simulink model "uart_xy_wiggler"  (R2018a)
settings: Solver=FixedStepDiscrete  StartTime=0.0  StopTime=inf  RelTol=1e-3
PreLoadFcn:
  | waijung.modelPreload; % Required for working with Waijung Blockset. Do not remove.
undefined symbols (not defined in the file or in its folder): HSEOSC, Link, LQFP144, ST, STM32F446ZE
libraries: simulink x10, commsynccomp2 x7, stm32f4_io_lib x3, dspstat3 x2, stm32f4_device_config_lib x1, dspbuff3 x1
(part 8 of 9)

== system uart_xy_wiggler/set_UART_VCflag/Set UART vc Flag=6 ==
  UART Command : Inport
  Enable : EnablePort
  Volatile Data Storage Write : S-Function  FunctionName=waijung_vdata_write  Parameters=storagename,varname,sampletime,sampletimestr,blockid,storagetype,storagetypestr  SFunctionDeploymentMode=off  EnableBusSupport=off  mask(waijung_vdata_write){storagename=CircleR, varname=VolatileDataStorage7_CircleR, sampletime=.01, sampletimestr=-1, blockid=set_UART_VCflagSetUARTvcFlag6VolatileDataStorageWrite, storagetype=double, storagetypestr=double}
      mask prompts: storagename "Storage Name"; varname "Variable name"; sampletime "Sample time (sec)"; sampletimestr "Compiled sample time (sec) in string"; storagetype "Data type"; storagetypestr "Data type string"
      mask help: This block implements write data to a buffer.
      mask init:
      | waijung_vdata_write_callback('init');
      mask Help: web(fullfile(waijungdocroot,'Volatile_Data_Storage_Write.htm'))
      mask TypeOptions storagename: ab3 | ab1 | ab2 | ab4 | ab5 | ab6 | ab7 | ab8 | ab9 | ab10 | Ays | Ayc | Axs | A_Laser | LissaFreq | Axc | Laser | vcx | flag | CircleFlag | CircleFrequency | vcy | CircleR
      mask Callback storagename: waijung_vdata_write_callback('storagename');
      mask Callback varname: waijung_vdata_write_callback('varname');
      mask Callback sampletime: waijung_vdata_write_callback('sampletime');
      mask Callback sampletimestr: waijung_vdata_write_callback('sampletimestr');
      mask Callback blockid: waijung_vdata_write_callback('blockid');
      mask Callback storagetype: waijung_vdata_write_callback('storagetype');
      mask Display: text(0.95, 0.5, 'Buffer: CircleR','ver','middle','hor','right');port_label('input',1,'D1(double)')
  wires:
  UART Command/1 -> Volatile Data Storage Write/1

== system uart_xy_wiggler/set_UART_VCflag/flag_setting ==
  In1 : Inport
  Enable : EnablePort
  Data Type Conversion : DataTypeConversion
  Volatile Data Storage Write : S-Function  FunctionName=waijung_vdata_write  Parameters=storagename,varname,sampletime,sampletimestr,blockid,storagetype,storagetypestr  SFunctionDeploymentMode=off  EnableBusSupport=off  mask(waijung_vdata_write){storagename=flag, varname=VolatileDataStorage3_flag, sampletime=-1, sampletimestr=-1, blockid=set_UART_VCflagflag_settingVolatileDataStorageWrite, storagetype=uint8, storagetypestr=uint8_t}
      mask prompts: storagename "Storage Name"; varname "Variable name"; sampletime "Sample time (sec)"; sampletimestr "Compiled sample time (sec) in string"; storagetype "Data type"; storagetypestr "Data type string"
      mask help: This block implements write data to a buffer.
      mask init:
      | waijung_vdata_write_callback('init');
      mask Help: web(fullfile(waijungdocroot,'Volatile_Data_Storage_Write.htm'))
      mask TypeOptions storagename: ab3 | ab1 | ab2 | ab4 | ab5 | ab6 | ab7 | ab8 | ab9 | ab10 | Ays | Ayc | Axs | A_Laser | LissaFreq | Axc | Laser | vcx | flag | CircleFlag | CircleFrequency | vcy | CircleR
      mask Callback storagename: waijung_vdata_write_callback('storagename');
      mask Callback varname: waijung_vdata_write_callback('varname');
      mask Callback sampletime: waijung_vdata_write_callback('sampletime');
      mask Callback sampletimestr: waijung_vdata_write_callback('sampletimestr');
      mask Callback blockid: waijung_vdata_write_callback('blockid');
      mask Callback storagetype: waijung_vdata_write_callback('storagetype');
      mask Display: text(0.95, 0.5, 'Buffer: flag','ver','middle','hor','right');port_label('input',1,'D1(uint8)')
  wires:
  Data Type Conversion/1 -> Volatile Data Storage Write/1
  In1/1 -> Data Type Conversion/1

== system uart_xy_wiggler/Circle/Calibration Y/Subsystem1 ==
  Mux2 : Mux  Inputs=5
  Volatile Data Storage Read10 : S-Function  FunctionName=waijung_vdata_read  Parameters=storagename,varname,sampletime,sampletimestr,blockid,storagetype,storagetypestr  SFunctionDeploymentMode=off  EnableBusSupport=off  mask(waijung_vdata_read){storagename=ab10, varname=CalibrationDataVolatileDataStorage8_ab10, sampletime=.01, sampletimestr=-1, blockid=CircleCalibrationYSubsystem1VolatileDataStorageRead10, storagetype=double, storagetypestr=double}
      mask prompts: storagename "Storage Name"; varname "Variable name"; sampletime "Sample time (sec)"; sampletimestr "Compiled sample time (sec) in string"; storagetype "Data type"; storagetypestr "Data type string"
      mask help: This block implements read data from a buffer.
      mask init:
      | waijung_vdata_read_callback('init');
      mask Help: web(fullfile(waijungdocroot,'Volatile_Data_Storage_Read.htm'))
      mask TypeOptions storagename: ab3 | ab1 | ab2 | ab4 | ab5 | ab6 | ab7 | ab8 | ab9 | ab10 | Ays | Ayc | Axs | A_Laser | LissaFreq | Axc | Laser | vcx | flag | CircleFlag | CircleFrequency | vcy | CircleR
      mask Callback storagename: waijung_vdata_read_callback('storagename');
      mask Callback varname: waijung_vdata_read_callback('varname');
      mask Callback sampletime: waijung_vdata_read_callback('sampletime');
      mask Callback sampletimestr: waijung_vdata_read_callback('sampletimestr');
      mask Callback blockid: waijung_vdata_read_callback('blockid');
      mask Callback storagetype: waijung_vdata_read_callback('storagetype');
      mask Display: text(0.05, 0.5, 'Buffer: ab10','ver','middle','hor','left');port_label('output',1,'D1(double)')
  Volatile Data Storage Read6 : S-Function  FunctionName=waijung_vdata_read  Parameters=storagename,varname,sampletime,sampletimestr,blockid,storagetype,storagetypestr  SFunctionDeploymentMode=off  EnableBusSupport=off  mask(waijung_vdata_read){storagename=ab7, varname=CalibrationDataVolatileDataStorage5_ab7, sampletime=.01, sampletimestr=-1, blockid=CircleCalibrationYSubsystem1VolatileDataStorageRead6, storagetype=double, storagetypestr=double}
      mask prompts: storagename "Storage Name"; varname "Variable name"; sampletime "Sample time (sec)"; sampletimestr "Compiled sample time (sec) in string"; storagetype "Data type"; storagetypestr "Data type string"
      mask help: This block implements read data from a buffer.
      mask init:
      | waijung_vdata_read_callback('init');
      mask Help: web(fullfile(waijungdocroot,'Volatile_Data_Storage_Read.htm'))
      mask TypeOptions storagename: ab3 | ab1 | ab2 | ab4 | ab5 | ab6 | ab7 | ab8 | ab9 | ab10 | Ays | Ayc | Axs | A_Laser | LissaFreq | Axc | Laser | vcx | flag | CircleFlag | CircleFrequency | vcy | CircleR
      mask Callback storagename: waijung_vdata_read_callback('storagename');
      mask Callback varname: waijung_vdata_read_callback('varname');
      mask Callback sampletime: waijung_vdata_read_callback('sampletime');
      mask Callback sampletimestr: waijung_vdata_read_callback('sampletimestr');
      mask Callback blockid: waijung_vdata_read_callback('blockid');
      mask Callback storagetype: waijung_vdata_read_callback('storagetype');
      mask Display: text(0.05, 0.5, 'Buffer: ab7','ver','middle','hor','left');port_label('output',1,'D1(double)')
  Volatile Data Storage Read7 : S-Function  FunctionName=waijung_vdata_read  Parameters=storagename,varname,sampletime,sampletimestr,blockid,storagetype,storagetypestr  SFunctionDeploymentMode=off  EnableBusSupport=off  mask(waijung_vdata_read){storagename=ab8, varname=CalibrationDataVolatileDataStorage6_ab8, sampletime=.01, sampletimestr=-1, blockid=CircleCalibrationYSubsystem1VolatileDataStorageRead7, storagetype=double, storagetypestr=double}
      mask prompts: storagename "Storage Name"; varname "Variable name"; sampletime "Sample time (sec)"; sampletimestr "Compiled sample time (sec) in string"; storagetype "Data type"; storagetypestr "Data type string"
      mask help: This block implements read data from a buffer.
      mask init:
      | waijung_vdata_read_callback('init');
      mask Help: web(fullfile(waijungdocroot,'Volatile_Data_Storage_Read.htm'))
      mask TypeOptions storagename: ab3 | ab1 | ab2 | ab4 | ab5 | ab6 | ab7 | ab8 | ab9 | ab10 | Ays | Ayc | Axs | A_Laser | LissaFreq | Axc | Laser | vcx | flag | CircleFlag | CircleFrequency | vcy | CircleR
      mask Callback storagename: waijung_vdata_read_callback('storagename');
      mask Callback varname: waijung_vdata_read_callback('varname');
      mask Callback sampletime: waijung_vdata_read_callback('sampletime');
      mask Callback sampletimestr: waijung_vdata_read_callback('sampletimestr');
      mask Callback blockid: waijung_vdata_read_callback('blockid');
      mask Callback storagetype: waijung_vdata_read_callback('storagetype');
      mask Display: text(0.05, 0.5, 'Buffer: ab8','ver','middle','hor','left');port_label('output',1,'D1(double)')
  Volatile Data Storage Read8 : S-Function  FunctionName=waijung_vdata_read  Parameters=storagename,varname,sampletime,sampletimestr,blockid,storagetype,storagetypestr  SFunctionDeploymentMode=off  EnableBusSupport=off  mask(waijung_vdata_read){storagename=ab9, varname=CalibrationDataVolatileDataStorage7_ab9, sampletime=.01, sampletimestr=-1, blockid=CircleCalibrationYSubsystem1VolatileDataStorageRead8, storagetype=double, storagetypestr=double}
      mask prompts: storagename "Storage Name"; varname "Variable name"; sampletime "Sample time (sec)"; sampletimestr "Compiled sample time (sec) in string"; storagetype "Data type"; storagetypestr "Data type string"
      mask help: This block implements read data from a buffer.
      mask init:
      | waijung_vdata_read_callback('init');
      mask Help: web(fullfile(waijungdocroot,'Volatile_Data_Storage_Read.htm'))
      mask TypeOptions storagename: ab3 | ab1 | ab2 | ab4 | ab5 | ab6 | ab7 | ab8 | ab9 | ab10 | Ays | Ayc | Axs | A_Laser | LissaFreq | Axc | Laser | vcx | flag | CircleFlag | CircleFrequency | vcy | CircleR
      mask Callback storagename: waijung_vdata_read_callback('storagename');
      mask Callback varname: waijung_vdata_read_callback('varname');
      mask Callback sampletime: waijung_vdata_read_callback('sampletime');
      mask Callback sampletimestr: waijung_vdata_read_callback('sampletimestr');
      mask Callback blockid: waijung_vdata_read_callback('blockid');
      mask Callback storagetype: waijung_vdata_read_callback('storagetype');
      mask Display: text(0.05, 0.5, 'Buffer: ab9','ver','middle','hor','left');port_label('output',1,'D1(double)')
  Volatile Data Storage Read9 : S-Function  FunctionName=waijung_vdata_read  Parameters=storagename,varname,sampletime,sampletimestr,blockid,storagetype,storagetypestr  SFunctionDeploymentMode=off  EnableBusSupport=off  mask(waijung_vdata_read){storagename=ab6, varname=CalibrationDataVolatileDataStorage4_ab6, sampletime=.01, sampletimestr=-1, blockid=CircleCalibrationYSubsystem1VolatileDataStorageRead9, storagetype=double, storagetypestr=double}
      mask prompts: storagename "Storage Name"; varname "Variable name"; sampletime "Sample time (sec)"; sampletimestr "Compiled sample time (sec) in string"; storagetype "Data type"; storagetypestr "Data type string"
      mask help: This block implements read data from a buffer.
      mask init:
      | waijung_vdata_read_callback('init');
      mask Help: web(fullfile(waijungdocroot,'Volatile_Data_Storage_Read.htm'))
      mask TypeOptions storagename: ab3 | ab1 | ab2 | ab4 | ab5 | ab6 | ab7 | ab8 | ab9 | ab10 | Ays | Ayc | Axs | A_Laser | LissaFreq | Axc | Laser | vcx | flag | CircleFlag | CircleFrequency | vcy | CircleR
      mask Callback storagename: waijung_vdata_read_callback('storagename');
      mask Callback varname: waijung_vdata_read_callback('varname');
      mask Callback sampletime: waijung_vdata_read_callback('sampletime');
      mask Callback sampletimestr: waijung_vdata_read_callback('sampletimestr');
      mask Callback blockid: waijung_vdata_read_callback('blockid');
      mask Callback storagetype: waijung_vdata_read_callback('storagetype');
      mask Display: text(0.05, 0.5, 'Buffer: ab6','ver','middle','hor','left');port_label('output',1,'D1(double)')
  Y Calibration Coeff : Outport
  wires:
  Volatile Data Storage Read10/1 -> Mux2/5
  Volatile Data Storage Read8/1 -> Mux2/4
  Volatile Data Storage Read6/1 -> Mux2/2
  Volatile Data Storage Read7/1 -> Mux2/3
  Mux2/1 -> Y Calibration Coeff/1
  Volatile Data Storage Read9/1 -> Mux2/1

== system uart_xy_wiggler/Circle/Calibrtaion X/Subsystem ==
  Mux : Mux  Inputs=5
  Volatile Data Storage Read1 : S-Function  FunctionName=waijung_vdata_read  Parameters=storagename,varname,sampletime,sampletimestr,blockid,storagetype,storagetypestr  SFunctionDeploymentMode=off  EnableBusSupport=off  mask(waijung_vdata_read){storagename=ab2, varname=CalibrationDataVolatileDataStorage12_ab2, sampletime=.01, sampletimestr=-1, blockid=CircleCalibrtaionXSubsystemVolatileDataStorageRead1, storagetype=double, storagetypestr=double}
      mask prompts: storagename "Storage Name"; varname "Variable name"; sampletime "Sample time (sec)"; sampletimestr "Compiled sample time (sec) in string"; storagetype "Data type"; storagetypestr "Data type string"
      mask help: This block implements read data from a buffer.
      mask init:
      | waijung_vdata_read_callback('init');
      mask Help: web(fullfile(waijungdocroot,'Volatile_Data_Storage_Read.htm'))
      mask TypeOptions storagename: ab3 | ab1 | ab2 | ab4 | ab5 | ab6 | ab7 | ab8 | ab9 | ab10 | Ays | Ayc | Axs | A_Laser | LissaFreq | Axc | Laser | vcx | flag | CircleFlag | CircleFrequency | vcy | CircleR
      mask Callback storagename: waijung_vdata_read_callback('storagename');
      mask Callback varname: waijung_vdata_read_callback('varname');
      mask Callback sampletime: waijung_vdata_read_callback('sampletime');
      mask Callback sampletimestr: waijung_vdata_read_callback('sampletimestr');
      mask Callback blockid: waijung_vdata_read_callback('blockid');
      mask Callback storagetype: waijung_vdata_read_callback('storagetype');
      mask Display: text(0.05, 0.5, 'Buffer: ab2','ver','middle','hor','left');port_label('output',1,'D1(double)')
  Volatile Data Storage Read2 : S-Function  FunctionName=waijung_vdata_read  Parameters=storagename,varname,sampletime,sampletimestr,blockid,storagetype,storagetypestr  SFunctionDeploymentMode=off  EnableBusSupport=off  mask(waijung_vdata_read){storagename=ab3, varname=CalibrationDataVolatileDataStorage1_ab3, sampletime=.01, sampletimestr=-1, blockid=CircleCalibrtaionXSubsystemVolatileDataStorageRead2, storagetype=double, storagetypestr=double}
      mask prompts: storagename "Storage Name"; varname "Variable name"; sampletime "Sample time (sec)"; sampletimestr "Compiled sample time (sec) in string"; storagetype "Data type"; storagetypestr "Data type string"
      mask help: This block implements read data from a buffer.
      mask init:
      | waijung_vdata_read_callback('init');
      mask Help: web(fullfile(waijungdocroot,'Volatile_Data_Storage_Read.htm'))
      mask TypeOptions storagename: ab3 | ab1 | ab2 | ab4 | ab5 | ab6 | ab7 | ab8 | ab9 | ab10 | Ays | Ayc | Axs | A_Laser | LissaFreq | Axc | Laser | vcx | flag | CircleFlag | CircleFrequency | vcy | CircleR
      mask Callback storagename: waijung_vdata_read_callback('storagename');
      mask Callback varname: waijung_vdata_read_callback('varname');
      mask Callback sampletime: waijung_vdata_read_callback('sampletime');
      mask Callback sampletimestr: waijung_vdata_read_callback('sampletimestr');
      mask Callback blockid: waijung_vdata_read_callback('blockid');
      mask Callback storagetype: waijung_vdata_read_callback('storagetype');
      mask Display: text(0.05, 0.5, 'Buffer: ab3','ver','middle','hor','left');port_label('output',1,'D1(double)')
  Volatile Data Storage Read3 : S-Function  FunctionName=waijung_vdata_read  Parameters=storagename,varname,sampletime,sampletimestr,blockid,storagetype,storagetypestr  SFunctionDeploymentMode=off  EnableBusSupport=off  mask(waijung_vdata_read){storagename=ab4, varname=CalibrationDataVolatileDataStorage2_ab4, sampletime=.01, sampletimestr=-1, blockid=CircleCalibrtaionXSubsystemVolatileDataStorageRead3, storagetype=double, storagetypestr=double}
      mask prompts: storagename "Storage Name"; varname "Variable name"; sampletime "Sample time (sec)"; sampletimestr "Compiled sample time (sec) in string"; storagetype "Data type"; storagetypestr "Data type string"
      mask help: This block implements read data from a buffer.
      mask init:
      | waijung_vdata_read_callback('init');
      mask Help: web(fullfile(waijungdocroot,'Volatile_Data_Storage_Read.htm'))
      mask TypeOptions storagename: ab3 | ab1 | ab2 | ab4 | ab5 | ab6 | ab7 | ab8 | ab9 | ab10 | Ays | Ayc | Axs | A_Laser | LissaFreq | Axc | Laser | vcx | flag | CircleFlag | CircleFrequency | vcy | CircleR
      mask Callback storagename: waijung_vdata_read_callback('storagename');
      mask Callback varname: waijung_vdata_read_callback('varname');
      mask Callback sampletime: waijung_vdata_read_callback('sampletime');
      mask Callback sampletimestr: waijung_vdata_read_callback('sampletimestr');
      mask Callback blockid: waijung_vdata_read_callback('blockid');
      mask Callback storagetype: waijung_vdata_read_callback('storagetype');
      mask Display: text(0.05, 0.5, 'Buffer: ab4','ver','middle','hor','left');port_label('output',1,'D1(double)')
  Volatile Data Storage Read4 : S-Function  FunctionName=waijung_vdata_read  Parameters=storagename,varname,sampletime,sampletimestr,blockid,storagetype,storagetypestr  SFunctionDeploymentMode=off  EnableBusSupport=off  mask(waijung_vdata_read){storagename=ab1, varname=CalibrationDataVolatileDataStorage11_ab1, sampletime=.01, sampletimestr=-1, blockid=CircleCalibrtaionXSubsystemVolatileDataStorageRead4, storagetype=double, storagetypestr=double}
      mask prompts: storagename "Storage Name"; varname "Variable name"; sampletime "Sample time (sec)"; sampletimestr "Compiled sample time (sec) in string"; storagetype "Data type"; storagetypestr "Data type string"
      mask help: This block implements read data from a buffer.
      mask init:
      | waijung_vdata_read_callback('init');
      mask Help: web(fullfile(waijungdocroot,'Volatile_Data_Storage_Read.htm'))
      mask TypeOptions storagename: ab3 | ab1 | ab2 | ab4 | ab5 | ab6 | ab7 | ab8 | ab9 | ab10 | Ays | Ayc | Axs | A_Laser | LissaFreq | Axc | Laser | vcx | flag | CircleFlag | CircleFrequency | vcy | CircleR
      mask Callback storagename: waijung_vdata_read_callback('storagename');
      mask Callback varname: waijung_vdata_read_callback('varname');
      mask Callback sampletime: waijung_vdata_read_callback('sampletime');
      mask Callback sampletimestr: waijung_vdata_read_callback('sampletimestr');
      mask Callback blockid: waijung_vdata_read_callback('blockid');
      mask Callback storagetype: waijung_vdata_read_callback('storagetype');
      mask Display: text(0.05, 0.5, 'Buffer: ab1','ver','middle','hor','left');port_label('output',1,'D1(double)')
  Volatile Data Storage Read5 : S-Function  FunctionName=waijung_vdata_read  Parameters=storagename,varname,sampletime,sampletimestr,blockid,storagetype,storagetypestr  SFunctionDeploymentMode=off  EnableBusSupport=off  mask(waijung_vdata_read){storagename=ab5, varname=CalibrationDataVolatileDataStorage3_ab5, sampletime=.01, sampletimestr=-1, blockid=CircleCalibrtaionXSubsystemVolatileDataStorageRead5, storagetype=double, storagetypestr=double}
      mask prompts: storagename "Storage Name"; varname "Variable name"; sampletime "Sample time (sec)"; sampletimestr "Compiled sample time (sec) in string"; storagetype "Data type"; storagetypestr "Data type string"
      mask help: This block implements read data from a buffer.
      mask init:
      | waijung_vdata_read_callback('init');
      mask Help: web(fullfile(waijungdocroot,'Volatile_Data_Storage_Read.htm'))
      mask TypeOptions storagename: ab3 | ab1 | ab2 | ab4 | ab5 | ab6 | ab7 | ab8 | ab9 | ab10 | Ays | Ayc | Axs | A_Laser | LissaFreq | Axc | Laser | vcx | flag | CircleFlag | CircleFrequency | vcy | CircleR
      mask Callback storagename: waijung_vdata_read_callback('storagename');
      mask Callback varname: waijung_vdata_read_callback('varname');
      mask Callback sampletime: waijung_vdata_read_callback('sampletime');
      mask Callback sampletimestr: waijung_vdata_read_callback('sampletimestr');
      mask Callback blockid: waijung_vdata_read_callback('blockid');
      mask Callback storagetype: waijung_vdata_read_callback('storagetype');
      mask Display: text(0.05, 0.5, 'Buffer: ab5','ver','middle','hor','left');port_label('output',1,'D1(double)')
  X Calibration Coeff : Outport
  wires:
  Volatile Data Storage Read4/1 -> Mux/1
  Volatile Data Storage Read1/1 -> Mux/2
  Volatile Data Storage Read2/1 -> Mux/3
  Volatile Data Storage Read3/1 -> Mux/4
  Volatile Data Storage Read5/1 -> Mux/5
  Mux/1 -> X Calibration Coeff/1

== system uart_xy_wiggler/Lissajous/Calibration Y/Subsystem1 ==
  Mux2 : Mux  Inputs=5
  Volatile Data Storage Read10 : S-Function  FunctionName=waijung_vdata_read  Parameters=storagename,varname,sampletime,sampletimestr,blockid,storagetype,storagetypestr  SFunctionDeploymentMode=off  EnableBusSupport=off  mask(waijung_vdata_read){storagename=ab10, varname=CalibrationDataVolatileDataStorage8_ab10, sampletime=.01, sampletimestr=-1, blockid=LissajousCalibrationYSubsystem1VolatileDataStorageRead10, storagetype=double, storagetypestr=double}
      mask prompts: storagename "Storage Name"; varname "Variable name"; sampletime "Sample time (sec)"; sampletimestr "Compiled sample time (sec) in string"; storagetype "Data type"; storagetypestr "Data type string"
      mask help: This block implements read data from a buffer.
      mask init:
      | waijung_vdata_read_callback('init');
      mask Help: web(fullfile(waijungdocroot,'Volatile_Data_Storage_Read.htm'))
      mask TypeOptions storagename: ab3 | ab1 | ab2 | ab4 | ab5 | ab6 | ab7 | ab8 | ab9 | ab10 | Ays | Ayc | Axs | A_Laser | LissaFreq | Axc | Laser | vcx | flag | CircleFlag | CircleFrequency | vcy | CircleR
      mask Callback storagename: waijung_vdata_read_callback('storagename');
      mask Callback varname: waijung_vdata_read_callback('varname');
      mask Callback sampletime: waijung_vdata_read_callback('sampletime');
      mask Callback sampletimestr: waijung_vdata_read_callback('sampletimestr');
      mask Callback blockid: waijung_vdata_read_callback('blockid');
      mask Callback storagetype: waijung_vdata_read_callback('storagetype');
      mask Display: text(0.05, 0.5, 'Buffer: ab10','ver','middle','hor','left');port_label('output',1,'D1(double)')
  Volatile Data Storage Read6 : S-Function  FunctionName=waijung_vdata_read  Parameters=storagename,varname,sampletime,sampletimestr,blockid,storagetype,storagetypestr  SFunctionDeploymentMode=off  EnableBusSupport=off  mask(waijung_vdata_read){storagename=ab7, varname=CalibrationDataVolatileDataStorage5_ab7, sampletime=.01, sampletimestr=-1, blockid=LissajousCalibrationYSubsystem1VolatileDataStorageRead6, storagetype=double, storagetypestr=double}
      mask prompts: storagename "Storage Name"; varname "Variable name"; sampletime "Sample time (sec)"; sampletimestr "Compiled sample time (sec) in string"; storagetype "Data type"; storagetypestr "Data type string"
      mask help: This block implements read data from a buffer.
      mask init:
      | waijung_vdata_read_callback('init');
      mask Help: web(fullfile(waijungdocroot,'Volatile_Data_Storage_Read.htm'))
      mask TypeOptions storagename: ab3 | ab1 | ab2 | ab4 | ab5 | ab6 | ab7 | ab8 | ab9 | ab10 | Ays | Ayc | Axs | A_Laser | LissaFreq | Axc | Laser | vcx | flag | CircleFlag | CircleFrequency | vcy | CircleR
      mask Callback storagename: waijung_vdata_read_callback('storagename');
      mask Callback varname: waijung_vdata_read_callback('varname');
      mask Callback sampletime: waijung_vdata_read_callback('sampletime');
      mask Callback sampletimestr: waijung_vdata_read_callback('sampletimestr');
      mask Callback blockid: waijung_vdata_read_callback('blockid');
      mask Callback storagetype: waijung_vdata_read_callback('storagetype');
      mask Display: text(0.05, 0.5, 'Buffer: ab7','ver','middle','hor','left');port_label('output',1,'D1(double)')
  Volatile Data Storage Read7 : S-Function  FunctionName=waijung_vdata_read  Parameters=storagename,varname,sampletime,sampletimestr,blockid,storagetype,storagetypestr  SFunctionDeploymentMode=off  EnableBusSupport=off  mask(waijung_vdata_read){storagename=ab8, varname=CalibrationDataVolatileDataStorage6_ab8, sampletime=.01, sampletimestr=-1, blockid=LissajousCalibrationYSubsystem1VolatileDataStorageRead7, storagetype=double, storagetypestr=double}
      mask prompts: storagename "Storage Name"; varname "Variable name"; sampletime "Sample time (sec)"; sampletimestr "Compiled sample time (sec) in string"; storagetype "Data type"; storagetypestr "Data type string"
      mask help: This block implements read data from a buffer.
      mask init:
      | waijung_vdata_read_callback('init');
      mask Help: web(fullfile(waijungdocroot,'Volatile_Data_Storage_Read.htm'))
      mask TypeOptions storagename: ab3 | ab1 | ab2 | ab4 | ab5 | ab6 | ab7 | ab8 | ab9 | ab10 | Ays | Ayc | Axs | A_Laser | LissaFreq | Axc | Laser | vcx | flag | CircleFlag | CircleFrequency | vcy | CircleR
      mask Callback storagename: waijung_vdata_read_callback('storagename');
      mask Callback varname: waijung_vdata_read_callback('varname');
      mask Callback sampletime: waijung_vdata_read_callback('sampletime');
      mask Callback sampletimestr: waijung_vdata_read_callback('sampletimestr');
      mask Callback blockid: waijung_vdata_read_callback('blockid');
      mask Callback storagetype: waijung_vdata_read_callback('storagetype');
      mask Display: text(0.05, 0.5, 'Buffer: ab8','ver','middle','hor','left');port_label('output',1,'D1(double)')
  Volatile Data Storage Read8 : S-Function  FunctionName=waijung_vdata_read  Parameters=storagename,varname,sampletime,sampletimestr,blockid,storagetype,storagetypestr  SFunctionDeploymentMode=off  EnableBusSupport=off  mask(waijung_vdata_read){storagename=ab9, varname=CalibrationDataVolatileDataStorage7_ab9, sampletime=.01, sampletimestr=-1, blockid=LissajousCalibrationYSubsystem1VolatileDataStorageRead8, storagetype=double, storagetypestr=double}
      mask prompts: storagename "Storage Name"; varname "Variable name"; sampletime "Sample time (sec)"; sampletimestr "Compiled sample time (sec) in string"; storagetype "Data type"; storagetypestr "Data type string"
      mask help: This block implements read data from a buffer.
      mask init:
      | waijung_vdata_read_callback('init');
      mask Help: web(fullfile(waijungdocroot,'Volatile_Data_Storage_Read.htm'))
      mask TypeOptions storagename: ab3 | ab1 | ab2 | ab4 | ab5 | ab6 | ab7 | ab8 | ab9 | ab10 | Ays | Ayc | Axs | A_Laser | LissaFreq | Axc | Laser | vcx | flag | CircleFlag | CircleFrequency | vcy | CircleR
      mask Callback storagename: waijung_vdata_read_callback('storagename');
      mask Callback varname: waijung_vdata_read_callback('varname');
      mask Callback sampletime: waijung_vdata_read_callback('sampletime');
      mask Callback sampletimestr: waijung_vdata_read_callback('sampletimestr');
      mask Callback blockid: waijung_vdata_read_callback('blockid');
      mask Callback storagetype: waijung_vdata_read_callback('storagetype');
      mask Display: text(0.05, 0.5, 'Buffer: ab9','ver','middle','hor','left');port_label('output',1,'D1(double)')
  Volatile Data Storage Read9 : S-Function  FunctionName=waijung_vdata_read  Parameters=storagename,varname,sampletime,sampletimestr,blockid,storagetype,storagetypestr  SFunctionDeploymentMode=off  EnableBusSupport=off  mask(waijung_vdata_read){storagename=ab6, varname=CalibrationDataVolatileDataStorage4_ab6, sampletime=.01, sampletimestr=-1, blockid=LissajousCalibrationYSubsystem1VolatileDataStorageRead9, storagetype=double, storagetypestr=double}
      mask prompts: storagename "Storage Name"; varname "Variable name"; sampletime "Sample time (sec)"; sampletimestr "Compiled sample time (sec) in string"; storagetype "Data type"; storagetypestr "Data type string"
      mask help: This block implements read data from a buffer.
      mask init:
      | waijung_vdata_read_callback('init');
      mask Help: web(fullfile(waijungdocroot,'Volatile_Data_Storage_Read.htm'))
      mask TypeOptions storagename: ab3 | ab1 | ab2 | ab4 | ab5 | ab6 | ab7 | ab8 | ab9 | ab10 | Ays | Ayc | Axs | A_Laser | LissaFreq | Axc | Laser | vcx | flag | CircleFlag | CircleFrequency | vcy | CircleR
      mask Callback storagename: waijung_vdata_read_callback('storagename');
      mask Callback varname: waijung_vdata_read_callback('varname');
      mask Callback sampletime: waijung_vdata_read_callback('sampletime');
      mask Callback sampletimestr: waijung_vdata_read_callback('sampletimestr');
      mask Callback blockid: waijung_vdata_read_callback('blockid');
      mask Callback storagetype: waijung_vdata_read_callback('storagetype');
      mask Display: text(0.05, 0.5, 'Buffer: ab6','ver','middle','hor','left');port_label('output',1,'D1(double)')
  Y Calibration Coeff : Outport
  wires:
  Volatile Data Storage Read10/1 -> Mux2/5
  Volatile Data Storage Read8/1 -> Mux2/4
  Volatile Data Storage Read6/1 -> Mux2/2
  Volatile Data Storage Read7/1 -> Mux2/3
  Mux2/1 -> Y Calibration Coeff/1
  Volatile Data Storage Read9/1 -> Mux2/1

== system uart_xy_wiggler/Lissajous/Calibrtaion X/Subsystem ==
  Mux : Mux  Inputs=5
  Volatile Data Storage Read1 : S-Function  FunctionName=waijung_vdata_read  Parameters=storagename,varname,sampletime,sampletimestr,blockid,storagetype,storagetypestr  SFunctionDeploymentMode=off  EnableBusSupport=off  mask(waijung_vdata_read){storagename=ab2, varname=CalibrationDataVolatileDataStorage12_ab2, sampletime=.01, sampletimestr=-1, blockid=LissajousCalibrtaionXSubsystemVolatileDataStorageRead1, storagetype=double, storagetypestr=double}
      mask prompts: storagename "Storage Name"; varname "Variable name"; sampletime "Sample time (sec)"; sampletimestr "Compiled sample time (sec) in string"; storagetype "Data type"; storagetypestr "Data type string"
      mask help: This block implements read data from a buffer.
      mask init:
      | waijung_vdata_read_callback('init');
      mask Help: web(fullfile(waijungdocroot,'Volatile_Data_Storage_Read.htm'))
      mask TypeOptions storagename: ab3 | ab1 | ab2 | ab4 | ab5 | ab6 | ab7 | ab8 | ab9 | ab10 | Ays | Ayc | Axs | A_Laser | LissaFreq | Axc | Laser | vcx | flag | CircleFlag | CircleFrequency | vcy | CircleR
      mask Callback storagename: waijung_vdata_read_callback('storagename');
      mask Callback varname: waijung_vdata_read_callback('varname');
      mask Callback sampletime: waijung_vdata_read_callback('sampletime');
      mask Callback sampletimestr: waijung_vdata_read_callback('sampletimestr');
      mask Callback blockid: waijung_vdata_read_callback('blockid');
      mask Callback storagetype: waijung_vdata_read_callback('storagetype');
      mask Display: text(0.05, 0.5, 'Buffer: ab2','ver','middle','hor','left');port_label('output',1,'D1(double)')
  Volatile Data Storage Read2 : S-Function  FunctionName=waijung_vdata_read  Parameters=storagename,varname,sampletime,sampletimestr,blockid,storagetype,storagetypestr  SFunctionDeploymentMode=off  EnableBusSupport=off  mask(waijung_vdata_read){storagename=ab3, varname=CalibrationDataVolatileDataStorage1_ab3, sampletime=.01, sampletimestr=-1, blockid=LissajousCalibrtaionXSubsystemVolatileDataStorageRead2, storagetype=double, storagetypestr=double}
      mask prompts: storagename "Storage Name"; varname "Variable name"; sampletime "Sample time (sec)"; sampletimestr "Compiled sample time (sec) in string"; storagetype "Data type"; storagetypestr "Data type string"
      mask help: This block implements read data from a buffer.
      mask init:
      | waijung_vdata_read_callback('init');
      mask Help: web(fullfile(waijungdocroot,'Volatile_Data_Storage_Read.htm'))
      mask TypeOptions storagename: ab3 | ab1 | ab2 | ab4 | ab5 | ab6 | ab7 | ab8 | ab9 | ab10 | Ays | Ayc | Axs | A_Laser | LissaFreq | Axc | Laser | vcx | flag | CircleFlag | CircleFrequency | vcy | CircleR
      mask Callback storagename: waijung_vdata_read_callback('storagename');
      mask Callback varname: waijung_vdata_read_callback('varname');
      mask Callback sampletime: waijung_vdata_read_callback('sampletime');
      mask Callback sampletimestr: waijung_vdata_read_callback('sampletimestr');
      mask Callback blockid: waijung_vdata_read_callback('blockid');
      mask Callback storagetype: waijung_vdata_read_callback('storagetype');
      mask Display: text(0.05, 0.5, 'Buffer: ab3','ver','middle','hor','left');port_label('output',1,'D1(double)')
  Volatile Data Storage Read3 : S-Function  FunctionName=waijung_vdata_read  Parameters=storagename,varname,sampletime,sampletimestr,blockid,storagetype,storagetypestr  SFunctionDeploymentMode=off  EnableBusSupport=off  mask(waijung_vdata_read){storagename=ab4, varname=CalibrationDataVolatileDataStorage2_ab4, sampletime=.01, sampletimestr=-1, blockid=LissajousCalibrtaionXSubsystemVolatileDataStorageRead3, storagetype=double, storagetypestr=double}
      mask prompts: storagename "Storage Name"; varname "Variable name"; sampletime "Sample time (sec)"; sampletimestr "Compiled sample time (sec) in string"; storagetype "Data type"; storagetypestr "Data type string"
      mask help: This block implements read data from a buffer.
      mask init:
      | waijung_vdata_read_callback('init');
      mask Help: web(fullfile(waijungdocroot,'Volatile_Data_Storage_Read.htm'))
      mask TypeOptions storagename: ab3 | ab1 | ab2 | ab4 | ab5 | ab6 | ab7 | ab8 | ab9 | ab10 | Ays | Ayc | Axs | A_Laser | LissaFreq | Axc | Laser | vcx | flag | CircleFlag | CircleFrequency | vcy | CircleR
      mask Callback storagename: waijung_vdata_read_callback('storagename');
      mask Callback varname: waijung_vdata_read_callback('varname');
      mask Callback sampletime: waijung_vdata_read_callback('sampletime');
      mask Callback sampletimestr: waijung_vdata_read_callback('sampletimestr');
      mask Callback blockid: waijung_vdata_read_callback('blockid');
      mask Callback storagetype: waijung_vdata_read_callback('storagetype');
      mask Display: text(0.05, 0.5, 'Buffer: ab4','ver','middle','hor','left');port_label('output',1,'D1(double)')
  Volatile Data Storage Read4 : S-Function  FunctionName=waijung_vdata_read  Parameters=storagename,varname,sampletime,sampletimestr,blockid,storagetype,storagetypestr  SFunctionDeploymentMode=off  EnableBusSupport=off  mask(waijung_vdata_read){storagename=ab1, varname=CalibrationDataVolatileDataStorage11_ab1, sampletime=.01, sampletimestr=-1, blockid=LissajousCalibrtaionXSubsystemVolatileDataStorageRead4, storagetype=double, storagetypestr=double}
      mask prompts: storagename "Storage Name"; varname "Variable name"; sampletime "Sample time (sec)"; sampletimestr "Compiled sample time (sec) in string"; storagetype "Data type"; storagetypestr "Data type string"
      mask help: This block implements read data from a buffer.
      mask init:
      | waijung_vdata_read_callback('init');
      mask Help: web(fullfile(waijungdocroot,'Volatile_Data_Storage_Read.htm'))
      mask TypeOptions storagename: ab3 | ab1 | ab2 | ab4 | ab5 | ab6 | ab7 | ab8 | ab9 | ab10 | Ays | Ayc | Axs | A_Laser | LissaFreq | Axc | Laser | vcx | flag | CircleFlag | CircleFrequency | vcy | CircleR
      mask Callback storagename: waijung_vdata_read_callback('storagename');
      mask Callback varname: waijung_vdata_read_callback('varname');
      mask Callback sampletime: waijung_vdata_read_callback('sampletime');
      mask Callback sampletimestr: waijung_vdata_read_callback('sampletimestr');
      mask Callback blockid: waijung_vdata_read_callback('blockid');
      mask Callback storagetype: waijung_vdata_read_callback('storagetype');
      mask Display: text(0.05, 0.5, 'Buffer: ab1','ver','middle','hor','left');port_label('output',1,'D1(double)')
  Volatile Data Storage Read5 : S-Function  FunctionName=waijung_vdata_read  Parameters=storagename,varname,sampletime,sampletimestr,blockid,storagetype,storagetypestr  SFunctionDeploymentMode=off  EnableBusSupport=off  mask(waijung_vdata_read){storagename=ab5, varname=CalibrationDataVolatileDataStorage3_ab5, sampletime=.01, sampletimestr=-1, blockid=LissajousCalibrtaionXSubsystemVolatileDataStorageRead5, storagetype=double, storagetypestr=double}
      mask prompts: storagename "Storage Name"; varname "Variable name"; sampletime "Sample time (sec)"; sampletimestr "Compiled sample time (sec) in string"; storagetype "Data type"; storagetypestr "Data type string"
      mask help: This block implements read data from a buffer.
      mask init:
      | waijung_vdata_read_callback('init');
      mask Help: web(fullfile(waijungdocroot,'Volatile_Data_Storage_Read.htm'))
      mask TypeOptions storagename: ab3 | ab1 | ab2 | ab4 | ab5 | ab6 | ab7 | ab8 | ab9 | ab10 | Ays | Ayc | Axs | A_Laser | LissaFreq | Axc | Laser | vcx | flag | CircleFlag | CircleFrequency | vcy | CircleR
      mask Callback storagename: waijung_vdata_read_callback('storagename');
      mask Callback varname: waijung_vdata_read_callback('varname');
      mask Callback sampletime: waijung_vdata_read_callback('sampletime');
      mask Callback sampletimestr: waijung_vdata_read_callback('sampletimestr');
      mask Callback blockid: waijung_vdata_read_callback('blockid');
      mask Callback storagetype: waijung_vdata_read_callback('storagetype');
      mask Display: text(0.05, 0.5, 'Buffer: ab5','ver','middle','hor','left');port_label('output',1,'D1(double)')
  X Calibration Coeff : Outport
  wires:
  Volatile Data Storage Read4/1 -> Mux/1
  Volatile Data Storage Read1/1 -> Mux/2
  Volatile Data Storage Read2/1 -> Mux/3
  Volatile Data Storage Read3/1 -> Mux/4
  Volatile Data Storage Read5/1 -> Mux/5
  Mux/1 -> X Calibration Coeff/1

== system uart_xy_wiggler/set_UART_VCflag/Calibration Data Uart/Set UART vc Flag=1 ==
  UART Command : Inport
  Enable : EnablePort
  Volatile Data Storage Write : S-Function  FunctionName=waijung_vdata_write  Parameters=storagename,varname,sampletime,sampletimestr,blockid,storagetype,storagetypestr  SFunctionDeploymentMode=off  EnableBusSupport=off  mask(waijung_vdata_write){storagename=ab3, varname=CalibrationDataVolatileDataStorage1_ab3, sampletime=.01, sampletimestr=-1, blockid=set_UART_VCflagCalibrationDataUartSetUARTvcFlag1VolatileDataStorageWrite, storagetype=double, storagetypestr=double}
      mask prompts: storagename "Storage Name"; varname "Variable name"; sampletime "Sample time (sec)"; sampletimestr "Compiled sample time (sec) in string"; storagetype "Data type"; storagetypestr "Data type string"
      mask help: This block implements write data to a buffer.
      mask init:
      | waijung_vdata_write_callback('init');
      mask Help: web(fullfile(waijungdocroot,'Volatile_Data_Storage_Write.htm'))
      mask TypeOptions storagename: ab3 | ab1 | ab2 | ab4 | ab5 | ab6 | ab7 | ab8 | ab9 | ab10 | Ays | Ayc | Axs | A_Laser | LissaFreq | Axc | Laser | vcx | flag | CircleFlag | CircleFrequency | vcy | CircleR
      mask Callback storagename: waijung_vdata_write_callback('storagename');
      mask Callback varname: waijung_vdata_write_callback('varname');
      mask Callback sampletime: waijung_vdata_write_callback('sampletime');
      mask Callback sampletimestr: waijung_vdata_write_callback('sampletimestr');
      mask Callback blockid: waijung_vdata_write_callback('blockid');
      mask Callback storagetype: waijung_vdata_write_callback('storagetype');
      mask Display: text(0.95, 0.5, 'Buffer: ab3','ver','middle','hor','right');port_label('input',1,'D1(double)')
  wires:
  UART Command/1 -> Volatile Data Storage Write/1

== system uart_xy_wiggler/set_UART_VCflag/Calibration Data Uart/Set UART vc Flag=10 ==
  UART Command : Inport
  Enable : EnablePort
  Volatile Data Storage Write : S-Function  FunctionName=waijung_vdata_write  Parameters=storagename,varname,sampletime,sampletimestr,blockid,storagetype,storagetypestr  SFunctionDeploymentMode=off  EnableBusSupport=off  mask(waijung_vdata_write){storagename=ab1, varname=CalibrationDataVolatileDataStorage11_ab1, sampletime=.01, sampletimestr=-1, blockid=set_UART_VCflagCalibrationDataUartSetUARTvcFlag10VolatileDataStorageWrite, storagetype=double, storagetypestr=double}
      mask prompts: storagename "Storage Name"; varname "Variable name"; sampletime "Sample time (sec)"; sampletimestr "Compiled sample time (sec) in string"; storagetype "Data type"; storagetypestr "Data type string"
      mask help: This block implements write data to a buffer.
      mask init:
      | waijung_vdata_write_callback('init');
      mask Help: web(fullfile(waijungdocroot,'Volatile_Data_Storage_Write.htm'))
      mask TypeOptions storagename: ab3 | ab1 | ab2 | ab4 | ab5 | ab6 | ab7 | ab8 | ab9 | ab10 | Ays | Ayc | Axs | A_Laser | LissaFreq | Axc | Laser | vcx | flag | CircleFlag | CircleFrequency | vcy | CircleR
      mask Callback storagename: waijung_vdata_write_callback('storagename');
      mask Callback varname: waijung_vdata_write_callback('varname');
      mask Callback sampletime: waijung_vdata_write_callback('sampletime');
      mask Callback sampletimestr: waijung_vdata_write_callback('sampletimestr');
      mask Callback blockid: waijung_vdata_write_callback('blockid');
      mask Callback storagetype: waijung_vdata_write_callback('storagetype');
      mask Display: text(0.95, 0.5, 'Buffer: ab1','ver','middle','hor','right');port_label('input',1,'D1(double)')
  wires:
  UART Command/1 -> Volatile Data Storage Write/1

== system uart_xy_wiggler/set_UART_VCflag/Calibration Data Uart/Set UART vc Flag=11 ==
  UART Command : Inport
  Enable : EnablePort
  Volatile Data Storage Write : S-Function  FunctionName=waijung_vdata_write  Parameters=storagename,varname,sampletime,sampletimestr,blockid,storagetype,storagetypestr  SFunctionDeploymentMode=off  EnableBusSupport=off  mask(waijung_vdata_write){storagename=ab2, varname=CalibrationDataVolatileDataStorage12_ab2, sampletime=.01, sampletimestr=-1, blockid=set_UART_VCflagCalibrationDataUartSetUARTvcFlag11VolatileDataStorageWrite, storagetype=double, storagetypestr=double}
      mask prompts: storagename "Storage Name"; varname "Variable name"; sampletime "Sample time (sec)"; sampletimestr "Compiled sample time (sec) in string"; storagetype "Data type"; storagetypestr "Data type string"
      mask help: This block implements write data to a buffer.
      mask init:
      | waijung_vdata_write_callback('init');
      mask Help: web(fullfile(waijungdocroot,'Volatile_Data_Storage_Write.htm'))
      mask TypeOptions storagename: ab3 | ab1 | ab2 | ab4 | ab5 | ab6 | ab7 | ab8 | ab9 | ab10 | Ays | Ayc | Axs | A_Laser | LissaFreq | Axc | Laser | vcx | flag | CircleFlag | CircleFrequency | vcy | CircleR
      mask Callback storagename: waijung_vdata_write_callback('storagename');
      mask Callback varname: waijung_vdata_write_callback('varname');
      mask Callback sampletime: waijung_vdata_write_callback('sampletime');
      mask Callback sampletimestr: waijung_vdata_write_callback('sampletimestr');
      mask Callback blockid: waijung_vdata_write_callback('blockid');
      mask Callback storagetype: waijung_vdata_write_callback('storagetype');
      mask Display: text(0.95, 0.5, 'Buffer: ab2','ver','middle','hor','right');port_label('input',1,'D1(double)')
  wires:
  UART Command/1 -> Volatile Data Storage Write/1

== system uart_xy_wiggler/set_UART_VCflag/Calibration Data Uart/Set UART vc Flag=2 ==
  UART Command : Inport
  Enable : EnablePort
  Volatile Data Storage Write : S-Function  FunctionName=waijung_vdata_write  Parameters=storagename,varname,sampletime,sampletimestr,blockid,storagetype,storagetypestr  SFunctionDeploymentMode=off  EnableBusSupport=off  mask(waijung_vdata_write){storagename=ab4, varname=CalibrationDataVolatileDataStorage2_ab4, sampletime=.01, sampletimestr=-1, blockid=set_UART_VCflagCalibrationDataUartSetUARTvcFlag2VolatileDataStorageWrite, storagetype=double, storagetypestr=double}
      mask prompts: storagename "Storage Name"; varname "Variable name"; sampletime "Sample time (sec)"; sampletimestr "Compiled sample time (sec) in string"; storagetype "Data type"; storagetypestr "Data type string"
      mask help: This block implements write data to a buffer.
      mask init:
      | waijung_vdata_write_callback('init');
      mask Help: web(fullfile(waijungdocroot,'Volatile_Data_Storage_Write.htm'))
      mask TypeOptions storagename: ab3 | ab1 | ab2 | ab4 | ab5 | ab6 | ab7 | ab8 | ab9 | ab10 | Ays | Ayc | Axs | A_Laser | LissaFreq | Axc | Laser | vcx | flag | CircleFlag | CircleFrequency | vcy | CircleR
      mask Callback storagename: waijung_vdata_write_callback('storagename');
      mask Callback varname: waijung_vdata_write_callback('varname');
      mask Callback sampletime: waijung_vdata_write_callback('sampletime');
      mask Callback sampletimestr: waijung_vdata_write_callback('sampletimestr');
      mask Callback blockid: waijung_vdata_write_callback('blockid');
      mask Callback storagetype: waijung_vdata_write_callback('storagetype');
      mask Display: text(0.95, 0.5, 'Buffer: ab4','ver','middle','hor','right');port_label('input',1,'D1(double)')
  wires:
  UART Command/1 -> Volatile Data Storage Write/1

== system uart_xy_wiggler/set_UART_VCflag/Calibration Data Uart/Set UART vc Flag=3 ==
  UART Command : Inport
  Enable : EnablePort
  Volatile Data Storage Write : S-Function  FunctionName=waijung_vdata_write  Parameters=storagename,varname,sampletime,sampletimestr,blockid,storagetype,storagetypestr  SFunctionDeploymentMode=off  EnableBusSupport=off  mask(waijung_vdata_write){storagename=ab5, varname=CalibrationDataVolatileDataStorage3_ab5, sampletime=.01, sampletimestr=-1, blockid=set_UART_VCflagCalibrationDataUartSetUARTvcFlag3VolatileDataStorageWrite, storagetype=double, storagetypestr=double}
      mask prompts: storagename "Storage Name"; varname "Variable name"; sampletime "Sample time (sec)"; sampletimestr "Compiled sample time (sec) in string"; storagetype "Data type"; storagetypestr "Data type string"
      mask help: This block implements write data to a buffer.
      mask init:
      | waijung_vdata_write_callback('init');
      mask Help: web(fullfile(waijungdocroot,'Volatile_Data_Storage_Write.htm'))
      mask TypeOptions storagename: ab3 | ab1 | ab2 | ab4 | ab5 | ab6 | ab7 | ab8 | ab9 | ab10 | Ays | Ayc | Axs | A_Laser | LissaFreq | Axc | Laser | vcx | flag | CircleFlag | CircleFrequency | vcy | CircleR
      mask Callback storagename: waijung_vdata_write_callback('storagename');
      mask Callback varname: waijung_vdata_write_callback('varname');
      mask Callback sampletime: waijung_vdata_write_callback('sampletime');
      mask Callback sampletimestr: waijung_vdata_write_callback('sampletimestr');
      mask Callback blockid: waijung_vdata_write_callback('blockid');
      mask Callback storagetype: waijung_vdata_write_callback('storagetype');
      mask Display: text(0.95, 0.5, 'Buffer: ab5','ver','middle','hor','right');port_label('input',1,'D1(double)')
  wires:
  UART Command/1 -> Volatile Data Storage Write/1

== system uart_xy_wiggler/set_UART_VCflag/Calibration Data Uart/Set UART vc Flag=4 ==
  UART Command : Inport
  Enable : EnablePort
  Volatile Data Storage Write : S-Function  FunctionName=waijung_vdata_write  Parameters=storagename,varname,sampletime,sampletimestr,blockid,storagetype,storagetypestr  SFunctionDeploymentMode=off  EnableBusSupport=off  mask(waijung_vdata_write){storagename=ab8, varname=CalibrationDataVolatileDataStorage6_ab8, sampletime=.01, sampletimestr=-1, blockid=set_UART_VCflagCalibrationDataUartSetUARTvcFlag4VolatileDataStorageWrite, storagetype=double, storagetypestr=double}
      mask prompts: storagename "Storage Name"; varname "Variable name"; sampletime "Sample time (sec)"; sampletimestr "Compiled sample time (sec) in string"; storagetype "Data type"; storagetypestr "Data type string"
      mask help: This block implements write data to a buffer.
      mask init:
      | waijung_vdata_write_callback('init');
      mask Help: web(fullfile(waijungdocroot,'Volatile_Data_Storage_Write.htm'))
      mask TypeOptions storagename: ab3 | ab1 | ab2 | ab4 | ab5 | ab6 | ab7 | ab8 | ab9 | ab10 | Ays | Ayc | Axs | A_Laser | LissaFreq | Axc | Laser | vcx | flag | CircleFlag | CircleFrequency | vcy | CircleR
      mask Callback storagename: waijung_vdata_write_callback('storagename');
      mask Callback varname: waijung_vdata_write_callback('varname');
      mask Callback sampletime: waijung_vdata_write_callback('sampletime');
      mask Callback sampletimestr: waijung_vdata_write_callback('sampletimestr');
      mask Callback blockid: waijung_vdata_write_callback('blockid');
      mask Callback storagetype: waijung_vdata_write_callback('storagetype');
      mask Display: text(0.95, 0.5, 'Buffer: ab8','ver','middle','hor','right');port_label('input',1,'D1(double)')
  wires:
  UART Command/1 -> Volatile Data Storage Write/1
